simulink model "FULL_IM_HESS"  (R2017b)
settings: Solver=ode4  StartTime=0.0  StopTime=SIMULPARAM.T_end  FixedStep=SIMULPARAM.Ts  RelTol=1e-3  EnableMultiTasking=on
undefined symbols (not defined in the file): BAT, Bat_current_control, BATCURRENTCONTROL, CHAS, Chopper, d_current_control, DC_bus_voltage_control, DCBUSCONTROL, DCCAP, dCURRENTCONTROL, ENV, Flux_control, FLUXCONTROL, FLUXSTRATEGY, IM, L, q_current_control, qCURRENTCONTROL, SC, SC_current_control, SCCURRENTCONTROL, Speed_control, SPEEDCONTROL, STRATEGY, TRANS
libraries: simulink x3
(part 2 of 2)

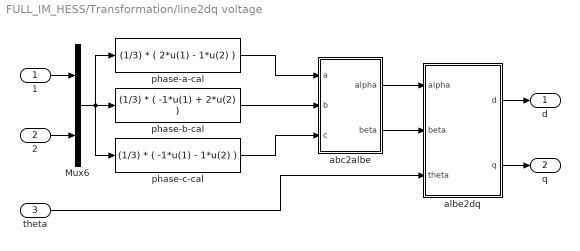
== system FULL_IM_HESS/Transformation/line2dq voltage ==
  1 : Inport
  2 : Inport  Port=2
  theta : Inport  Port=3
  Mux6 : Mux  Inputs=2
  abc2albe : Subsystem
  albe2dq : Subsystem
  phase-a-cal : Fcn  Expr=(1/3) * ( 2*u(1) - 1*u(2) )
  phase-b-cal : Fcn  Expr=(1/3) * ( -1*u(1) + 2*u(2) )
  phase-c-cal : Fcn  Expr=(1/3) * ( -1*u(1) - 1*u(2) )
  d : Outport
  q : Outport  Port=2
  wires:
  albe2dq/1(d) -> d/1
  albe2dq/2(q) -> q/1
  1/1 -> Mux6/1
  2/1 -> Mux6/2
  abc2albe/1(alpha) -> albe2dq/1(alpha)
  abc2albe/2(beta) -> albe2dq/2(beta)
  phase-b-cal/1 -> abc2albe/2(b)
  phase-a-cal/1 -> abc2albe/1(a)
  phase-c-cal/1 -> abc2albe/3(c)
  Mux6/1 -> phase-b-cal/1, phase-c-cal/1, phase-a-cal/1
  theta/1 -> albe2dq/3(theta)

== system FULL_IM_HESS/Vehicle speed controller/IP controller ==
  v_veh_meas : Inport
  v_veh_ref : Inport  Port=2
  Gain : Gain  Gain=SPEEDCONTROL.Kp_ip
  Gain1 : Gain  Gain=SPEEDCONTROL.Ki_ip
  Integrator : Integrator
  Sum1 : Sum  Inputs=-+
  Sum3 : Sum  Inputs=+-
  F_tran_ref : Outport
  wires:
  v_veh_ref/1 -> Sum1/2
  Gain/1 -> Sum3/2
  Integrator/1 -> Gain1/1
  v_veh_meas/1 -> Sum1/1, Gain/1
  Gain1/1 -> Sum3/1
  Sum3/1 -> F_tran_ref/1
  Sum1/1 -> Integrator/1

== system FULL_IM_HESS/Vehicle speed controller/PI controller ==
  v_veh_meas : Inport
  v_veh_ref : Inport  Port=2
  Gain : Gain  Gain=SPEEDCONTROL.Kp_pi
  Gain1 : Gain  Gain=SPEEDCONTROL.Ki_pi
  Integrator : Integrator
  Sum1 : Sum  Inputs=-+
  Sum3 : Sum
  F_tran_ref : Outport
  wires:
  Sum1/1 -> Gain/1, Integrator/1
  Sum3/1 -> F_tran_ref/1
  Gain1/1 -> Sum3/1
  v_veh_meas/1 -> Sum1/1
  Integrator/1 -> Gain1/1
  Gain/1 -> Sum3/2
  v_veh_ref/1 -> Sum1/2

== system FULL_IM_HESS/d-current controller/IP controller ==
  i_ds_meas : Inport
  i_ds_ref : Inport  Port=2
  Gain : Gain  Gain=dCURRENTCONTROL.Kp_ip
  Gain1 : Gain  Gain=dCURRENTCONTROL.Ki_ip
  Integrator : Integrator
  Sum : Sum  Inputs=+-
  Sum1 : Sum  Inputs=-+
  u_ds_arm : Outport
  wires:
  Gain1/1 -> Integrator/1
  i_ds_ref/1 -> Sum1/2
  i_ds_meas/1 -> Gain/1, Sum1/1
  Sum1/1 -> Gain1/1
  Sum/1 -> u_ds_arm/1
  Integrator/1 -> Sum/1
  Gain/1 -> Sum/2

== system FULL_IM_HESS/d-current controller/PI controller ==
  i_ds_meas : Inport
  i_ds_ref : Inport  Port=2
  Gain : Gain  Gain=dCURRENTCONTROL.Kp_pi
  Gain1 : Gain  Gain=dCURRENTCONTROL.Ki_pi
  Integrator : Integrator
  Sum : Sum
  Sum1 : Sum  Inputs=-+
  u_ds_arm : Outport
  wires:
  Gain/1 -> Sum/1
  Sum/1 -> u_ds_arm/1
  Sum1/1 -> Gain1/1, Gain/1
  i_ds_meas/1 -> Sum1/1
  Integrator/1 -> Sum/2
  i_ds_ref/1 -> Sum1/2
  Gain1/1 -> Integrator/1

== system FULL_IM_HESS/q-current controller/IP controller ==
  i_qs_meas : Inport
  i_qs_ref : Inport  Port=2
  Gain : Gain  Gain=qCURRENTCONTROL.Kp_ip
  Gain1 : Gain  Gain=qCURRENTCONTROL.Ki_ip
  Integrator : Integrator
  Sum : Sum  Inputs=+-
  Sum1 : Sum  Inputs=-+
  u_qs_arm : Outport
  wires:
  Gain1/1 -> Integrator/1
  i_qs_ref/1 -> Sum1/2
  i_qs_meas/1 -> Gain/1, Sum1/1
  Sum1/1 -> Gain1/1
  Sum/1 -> u_qs_arm/1
  Integrator/1 -> Sum/1
  Gain/1 -> Sum/2

== system FULL_IM_HESS/q-current controller/PI controller ==
  i_qs_meas : Inport
  i_qs_ref : Inport  Port=2
  Gain : Gain  Gain=qCURRENTCONTROL.Kp_pi
  Gain1 : Gain  Gain=qCURRENTCONTROL.Ki_pi
  Integrator : Integrator
  Sum : Sum
  Sum1 : Sum  Inputs=-+
  u_qs_arm : Outport
  wires:
  Gain/1 -> Sum/1
  Sum/1 -> u_qs_arm/1
  Sum1/1 -> Gain1/1, Gain/1
  i_qs_meas/1 -> Sum1/1
  Integrator/1 -> Sum/2
  i_qs_ref/1 -> Sum1/2
  Gain1/1 -> Integrator/1

== system FULL_IM_HESS/EMS/Conventional strategy/SC recharge logic ==
  i_tot_ref : Inport
  Abs : Abs
  Constant1 : Constant
  Relational Operator : RelationalOperator  Operator=<  OutDataTypeStr=boolean  RndMeth=Nearest
  Charge : Outport
  wires:
  Constant1/1 -> Relational Operator/2
  Abs/1 -> Relational Operator/1
  i_tot_ref/1 -> Abs/1
  Relational Operator/1 -> Charge/1

== system FULL_IM_HESS/EMS/Limitation/Limitation transition ==
  i_tot_meas : Inport
  i_ch_bat_ref_cal : Inport  Port=2
  u_sc_meas : Inport  Port=3
  1-D Lookup Table : Lookup_n-D  NumberOfTableDimensions=1  BreakpointsForDimension1=[SC.U_min SC.U_hi SC.U_max]  Table=[0 0 1]  InternalRulePriority=Speed  RndMeth=Simplest  InputSameDT=on
  1-D Lookup Table1 : Lookup_n-D  NumberOfTableDimensions=1  BreakpointsForDimension1=[SC.U_min SC.U_lo SC.U_max]  Table=[1 0 0]  InternalRulePriority=Speed  RndMeth=Simplest  InputSameDT=on
  Add1 : Sum  Inputs=+-
  Switch1 : Switch
  k_d : Outport
  wires:
  1-D Lookup Table1/1 -> Switch1/1
  i_ch_bat_ref_cal/1 -> Add1/2
  i_tot_meas/1 -> Add1/1
  Switch1/1 -> k_d/1
  Add1/1 -> Switch1/2
  u_sc_meas/1 -> 1-D Lookup Table/1, 1-D Lookup Table1/1
  1-D Lookup Table/1 -> Switch1/3

== system FULL_IM_HESS/Inverse trans/dq2line voltage/albe2abc ==
  alpha : Inport
  beta : Inport  Port=2
  Mux : Mux  Inputs=2
  a-cal : Fcn  Expr=u(1)
  b-cal : Fcn  Expr=(-u(1) + sqrt(3)*u(2))/2
  c-cal : Fcn  Expr=(-u(1) - sqrt(3)*u(2))/2
  a : Outport
  b : Outport  Port=2
  c : Outport  Port=3
  wires:
  alpha/1 -> Mux/1
  beta/1 -> Mux/2
  Mux/1 -> a-cal/1, b-cal/1, c-cal/1
  a-cal/1 -> a/1
  b-cal/1 -> b/1
  c-cal/1 -> c/1

== system FULL_IM_HESS/Inverse trans/dq2line voltage/dq2albe ==
  d : Inport
  q : Inport  Port=2
  theta : Inport  Port=3
  Mux : Mux  Inputs=3
  al-cal : Fcn  Expr=cos(u(3))*u(1) - sin(u(3))*u(2)
  be-cal : Fcn  Expr=sin(u(3))*u(1) + cos(u(3))*u(2)
  alpha : Outport
  beta : Outport  Port=2
  wires:
  Mux/1 -> al-cal/1, be-cal/1
  d/1 -> Mux/1
  al-cal/1 -> alpha/1
  q/1 -> Mux/2
  be-cal/1 -> beta/1
  theta/1 -> Mux/3

== system FULL_IM_HESS/Trans/current line2dq/abc2albe ==
  a : Inport
  b : Inport  Port=2
  c : Inport  Port=3
  Mux : Mux  Inputs=3
  al-cal : Fcn  Expr=(2/3)*u(1) - (1/3)*u(2) - (1/3)*u(3)
  q-cal : Fcn  Expr=0*u(1) + (1/sqrt(3))*(u(2) - u(3))
  alpha : Outport
  beta : Outport  Port=2
  wires:
  q-cal/1 -> beta/1
  al-cal/1 -> alpha/1
  Mux/1 -> q-cal/1, al-cal/1
  c/1 -> Mux/3
  b/1 -> Mux/2
  a/1 -> Mux/1

== system FULL_IM_HESS/Trans/current line2dq/albe2dq ==
  alpha : Inport
  beta : Inport  Port=2
  theta : Inport  Port=3
  Mux : Mux  Inputs=3
  d-cal : Fcn  Expr=cos(u(3))*u(1) + sin(u(3))*u(2)
  q-cal : Fcn  Expr=-sin(u(3))*u(1) + cos(u(3))*u(2)
  d : Outport
  q : Outport  Port=2
  wires:
  q-cal/1 -> q/1
  d-cal/1 -> d/1
  Mux/1 -> q-cal/1, d-cal/1
  theta/1 -> Mux/3
  beta/1 -> Mux/2
  alpha/1 -> Mux/1

== system FULL_IM_HESS/Transformation/dq2line current/albe2abc ==
  alpha : Inport
  beta : Inport  Port=2
  Mux : Mux  Inputs=2
  a-cal : Fcn  Expr=u(1)
  b-cal : Fcn  Expr=(-u(1) + sqrt(3)*u(2))/2
  c-cal : Fcn  Expr=(-u(1) - sqrt(3)*u(2))/2
  a : Outport
  b : Outport  Port=2
  c : Outport  Port=3
  wires:
  alpha/1 -> Mux/1
  beta/1 -> Mux/2
  Mux/1 -> b-cal/1, c-cal/1, a-cal/1
  a-cal/1 -> a/1
  b-cal/1 -> b/1
  c-cal/1 -> c/1

== system FULL_IM_HESS/Transformation/dq2line current/dq2albe ==
  d : Inport
  q : Inport  Port=2
  theta : Inport  Port=3
  Mux : Mux  Inputs=3
  al-cal : Fcn  Expr=cos(u(3))*u(1) - sin(u(3))*u(2)
  be-cal : Fcn  Expr=sin(u(3))*u(1) + cos(u(3))*u(2)
  alpha : Outport
  beta : Outport  Port=2
  wires:
  Mux/1 -> al-cal/1, be-cal/1
  d/1 -> Mux/1
  al-cal/1 -> alpha/1
  q/1 -> Mux/2
  be-cal/1 -> beta/1
  theta/1 -> Mux/3

== system FULL_IM_HESS/Transformation/line2dq voltage/abc2albe ==
  a : Inport
  b : Inport  Port=2
  c : Inport  Port=3
  Mux : Mux  Inputs=3
  al-cal : Fcn  Expr=(2/3)*u(1) - (1/3)*u(2) - (1/3)*u(3)
  q-cal : Fcn  Expr=0*u(1) + (1/sqrt(3))*(u(2) - u(3))
  alpha : Outport
  beta : Outport  Port=2
  wires:
  q-cal/1 -> beta/1
  al-cal/1 -> alpha/1
  Mux/1 -> q-cal/1, al-cal/1
  c/1 -> Mux/3
  b/1 -> Mux/2
  a/1 -> Mux/1

== system FULL_IM_HESS/Transformation/line2dq voltage/albe2dq ==
  alpha : Inport
  beta : Inport  Port=2
  theta : Inport  Port=3
  Mux : Mux  Inputs=3
  d-cal : Fcn  Expr=cos(u(3))*u(1) + sin(u(3))*u(2)
  q-cal : Fcn  Expr=-sin(u(3))*u(1) + cos(u(3))*u(2)
  d : Outport
  q : Outport  Port=2
  wires:
  q-cal/1 -> q/1
  d-cal/1 -> d/1
  Mux/1 -> q-cal/1, d-cal/1
  theta/1 -> Mux/3
  beta/1 -> Mux/2
  alpha/1 -> Mux/1
